simulink model "BaseEngineController_LS"  (Simulink 7.7)
settings: Solver=FixedStepDiscrete  StartTime=0.0  StopTime=10.0  RelTol=1e-3
PreLoadFcn:
  | try, eval([bdroot '_setup']); catch, eval('model_setup', ''); end
InitFcn:
  | try, eval([bdroot '_setup']); catch, eval('model_setup', ''); end
undefined symbols (not defined in the file): ECU555, High, motohawk_build_version, motohawk_trunc_name, motohawk_vardec_config_group, motohawk_vardec_path, True
libraries: MotoHawk_lib x1418, motohawk_control_primitives_lib x183, motohawk_engine_lib x32, simulink x21, motohawk_annotations_lib x9, AutoDoc_lib x8, simulink_extras x4, motohawk_ccp_examples_lib x1, motohawk_control_primitives_motoshare_lib x1
(part 12 of 27)

== system BaseEngineController_LS/Foreground/Control/Controller/Run/AC Control ==
  Sensors : Inport
  Trigger : TriggerPort  TriggerType=function-call
  AC Comp High Pressure : Subsystem  AncestorBlock=motohawk_control_primitives_lib/Hysterisis
      mask Display:
      | patch([0 0 1 1], [0 0.075 0.075 0], [230/255 0/255 0/255])
      | patch([0 0 1 1], [0.025 0.05 0.05 0.025], [150/255 0/255 0/255])
      | patch([0 0 1 1], [0 0.025 0.025 0], [0/255 0/255 0/255])
      | 
      | disp('HYSTERISIS')
  AC Comp Low Pressure : Subsystem  AncestorBlock=motohawk_control_primitives_lib/Hysterisis
      mask Display:
      | patch([0 0 1 1], [0 0.075 0.075 0], [230/255 0/255 0/255])
      | patch([0 0 1 1], [0.025 0.05 0.05 0.025], [150/255 0/255 0/255])
      | patch([0 0 1 1], [0 0.025 0.025 0], [0/255 0/255 0/255])
      | 
      | disp('HYSTERISIS')
  AC Comp Overspeed : Subsystem  AncestorBlock=motohawk_control_primitives_lib/Hysterisis
      mask Display:
      | patch([0 0 1 1], [0 0.075 0.075 0], [230/255 0/255 0/255])
      | patch([0 0 1 1], [0.025 0.05 0.05 0.025], [150/255 0/255 0/255])
      | patch([0 0 1 1], [0 0.025 0.025 0], [0/255 0/255 0/255])
      | 
      | disp('HYSTERISIS')
  AC Comp Overspeed1 : Subsystem  AncestorBlock=motohawk_control_primitives_lib/Hysterisis
      mask Display:
      | patch([0 0 1 1], [0 0.075 0.075 0], [230/255 0/255 0/255])
      | patch([0 0 1 1], [0.025 0.05 0.05 0.025], [150/255 0/255 0/255])
      | patch([0 0 1 1], [0 0.025 0.025 0], [0/255 0/255 0/255])
      | 
      | disp('HYSTERISIS')
  AC Comp Underspeed : Subsystem  AncestorBlock=motohawk_control_primitives_lib/Hysterisis
      mask Display:
      | patch([0 0 1 1], [0 0.075 0.075 0], [230/255 0/255 0/255])
      | patch([0 0 1 1], [0.025 0.05 0.05 0.025], [150/255 0/255 0/255])
      | patch([0 0 1 1], [0 0.025 0.025 0], [0/255 0/255 0/255])
      | 
      | disp('HYSTERISIS')
  AC Evap Temp Hyst : Subsystem  AncestorBlock=motohawk_control_primitives_lib/Hysterisis
      mask Display:
      | patch([0 0 1 1], [0 0.075 0.075 0], [230/255 0/255 0/255])
      | patch([0 0 1 1], [0.025 0.05 0.05 0.025], [150/255 0/255 0/255])
      | patch([0 0 1 1], [0 0.025 0.025 0], [0/255 0/255 0/255])
      | 
      | disp('HYSTERISIS')
  Bus Selector : BusSelector  OutputSignals=Raw.Digital.ACSw,Raw.NonLinearSensors.EVAP
  Bus Selector1 : BusSelector  OutputSignals=Raw.RPM
  Bus Selector2 : BusSelector  OutputSignals=RawProcessed.TPS
  Bus Selector3 : BusSelector  OutputSignals=Raw.LinearSensors.ACPres
  Bus Selector4 : BusSelector  OutputSignals=RawProcessed.TimeSinceRun
  Data Type Conversion : DataTypeConversion  OutDataTypeStr=uint16
  Data Type Conversion1 : DataTypeConversion  OutDataTypeStr=uint16
  Data Type Conversion2 : DataTypeConversion  OutDataTypeStr=uint16
  Logical Operator : Logic  Inputs=8  AllPortsSameDT=off  OutDataTypeStr=boolean
  Logical Operator{1..2,4,6} (4 alike) : Logic  Operator=NOT  AllPortsSameDT=off  OutDataTypeStr=boolean
  Logical Operator3 : Logic  AllPortsSameDT=off  OutDataTypeStr=boolean
  Relational Operator : RelationalOperator  OutDataTypeStr=boolean
  motohawk_calibration : MotoHawk_lib/Calibration & Probing Blocks/motohawk_calibration  nam='ACTempOn'  val=0  storage=Calibration  show_more=on  name_source=Use Parameter  data_type=double  read_level=1  write_level=1  ovr_cals=on  view_as=Number  enum_struct={'Disabled', 'Enabled'}  vector_style=Wide Row  use_help_units=off  help=''  units=''  use_header_enum=off  row_header_enum={}  col_header_enum={}  use_min_max=off  min_val=-inf  max_val=inf  use_precision=off  precision=''  gain=1  offset=0  exp=1  use_mototune_group=off  mototune_group=motohawk_vardec_path(gcb)
  motohawk_calibration1 : MotoHawk_lib/Calibration & Probing Blocks/motohawk_calibration  nam='ACSpdSlowOff'  val=200  storage=Calibration  show_more=on  name_source=Use Parameter  data_type=uint16  read_level=1  write_level=1  ovr_cals=on  view_as=Number  enum_struct={'Disabled', 'Enabled'}  vector_style=Wide Row  use_help_units=on  help='Engine speed at which the compressor turns off at low side'  units='RPM'  use_header_enum=off  row_header_enum={}  col_header_enum={}  use_min_max=off  min_val=-inf  max_val=inf  use_precision=off  precision=''  gain=1  offset=0  exp=1  use_mototune_group=off  mototune_group=motohawk_vardec_path(gcb)
  motohawk_calibration10 : MotoHawk_lib/Calibration & Probing Blocks/motohawk_calibration  nam='ACLowPresOff'  val=0  storage=Calibration  show_more=on  name_source=Use Parameter  data_type=uint16  read_level=1  write_level=1  ovr_cals=on  view_as=Number  enum_struct={'Disabled', 'Enabled'}  vector_style=Wide Row  use_help_units=off  help=''  units=''  use_header_enum=off  row_header_enum={}  col_header_enum={}  use_min_max=off  min_val=-inf  max_val=inf  use_precision=off  precision=''  gain=1  offset=0  exp=1  use_mototune_group=off  mototune_group=motohawk_vardec_path(gcb)
  motohawk_calibration11 : MotoHawk_lib/Calibration & Probing Blocks/motohawk_calibration  nam='ACHighPresOff'  val=0  storage=Calibration  show_more=on  name_source=Use Parameter  data_type=uint16  read_level=1  write_level=1  ovr_cals=on  view_as=Number  enum_struct={'Disabled', 'Enabled'}  vector_style=Wide Row  use_help_units=off  help=''  units=''  use_header_enum=off  row_header_enum={}  col_header_enum={}  use_min_max=off  min_val=-inf  max_val=inf  use_precision=off  precision=''  gain=1  offset=0  exp=1  use_mototune_group=off  mototune_group=motohawk_vardec_path(gcb)
  motohawk_calibration12 : MotoHawk_lib/Calibration & Probing Blocks/motohawk_calibration  nam='ACHighPresOn'  val=0  storage=Calibration  show_more=on  name_source=Use Parameter  data_type=uint16  read_level=1  write_level=1  ovr_cals=on  view_as=Number  enum_struct={'Disabled', 'Enabled'}  vector_style=Wide Row  use_help_units=off  help=''  units=''  use_header_enum=off  row_header_enum={}  col_header_enum={}  use_min_max=off  min_val=-inf  max_val=inf  use_precision=off  precision=''  gain=1  offset=0  exp=1  use_mototune_group=off  mototune_group=motohawk_vardec_path(gcb)
  motohawk_calibration2 : MotoHawk_lib/Calibration & Probing Blocks/motohawk_calibration  nam='ACSpdSlowOn'  val=400  storage=Calibration  show_more=on  name_source=Use Parameter  data_type=uint16  read_level=1  write_level=1  ovr_cals=on  view_as=Number  enum_struct={'Disabled', 'Enabled'}  vector_style=Wide Row  use_help_units=on  help='Engine speed at which the compressor turns on at low side'  units='RPM'  use_header_enum=off  row_header_enum={}  col_header_enum={}  use_min_max=off  min_val=-inf  max_val=inf  use_precision=off  precision=''  gain=1  offset=0  exp=1  use_mototune_group=off  mototune_group=motohawk_vardec_path(gcb)
  motohawk_calibration3 : MotoHawk_lib/Calibration & Probing Blocks/motohawk_calibration  nam='ACSpdFastOff'  val=4500  storage=Calibration  show_more=on  name_source=Use Parameter  data_type=uint16  read_level=1  write_level=1  ovr_cals=on  view_as=Number  enum_struct={'Disabled', 'Enabled'}  vector_style=Wide Row  use_help_units=on  help='Engine speed at which the compressor turns off at high side'  units='RPM'  use_header_enum=off  row_header_enum={}  col_header_enum={}  use_min_max=off  min_val=-inf  max_val=inf  use_precision=off  precision=''  gain=1  offset=0  exp=1  use_mototune_group=off  mototune_group=motohawk_vardec_path(gcb)
  motohawk_calibration4 : MotoHawk_lib/Calibration & Probing Blocks/motohawk_calibration  nam='ACSpdFastOn'  val=3000  storage=Calibration  show_more=on  name_source=Use Parameter  data_type=uint16  read_level=1  write_level=1  ovr_cals=on  view_as=Number  enum_struct={'Disabled', 'Enabled'}  vector_style=Wide Row  use_help_units=on  help='Engine speed at which the compressor turns on at high side'  units='RPM'  use_header_enum=off  row_header_enum={}  col_header_enum={}  use_min_max=off  min_val=-inf  max_val=inf  use_precision=off  precision=''  gain=1  offset=0  exp=1  use_mototune_group=off  mototune_group=motohawk_vardec_path(gcb)
  motohawk_calibration5 : MotoHawk_lib/Calibration & Probing Blocks/motohawk_calibration  nam='AC_TPSOff'  val=90  storage=Calibration  show_more=on  name_source=Use Parameter  data_type=uint16  read_level=1  write_level=1  ovr_cals=on  view_as=Number  enum_struct={'Disabled', 'Enabled'}  vector_style=Wide Row  use_help_units=on  help='Throttle position at which AC gets disengaged'  units='%'  use_header_enum=off  row_header_enum={}  col_header_enum={}  use_min_max=off  min_val=-inf  max_val=inf  use_precision=off  precision=''  gain=1  offset=0  exp=1  use_mototune_group=off  mototune_group=motohawk_vardec_path(gcb)
  motohawk_calibration6 : MotoHawk_lib/Calibration & Probing Blocks/motohawk_calibration  nam='AC_TPSOn'  val=80  storage=Calibration  show_more=on  name_source=Use Parameter  data_type=uint16  read_level=1  write_level=1  ovr_cals=on  view_as=Number  enum_struct={'Disabled', 'Enabled'}  vector_style=Wide Row  use_help_units=on  help='Throttle position at which AC gets engaged'  units='%'  use_header_enum=off  row_header_enum={}  col_header_enum={}  use_min_max=off  min_val=-inf  max_val=inf  use_precision=off  precision=''  gain=1  offset=0  exp=1  use_mototune_group=off  mototune_group=motohawk_vardec_path(gcb)
  motohawk_calibration7 : MotoHawk_lib/Calibration & Probing Blocks/motohawk_calibration  nam='ACTimeFromStartDelay'  val=3  storage=Calibration  show_more=on  name_source=Use Parameter  data_type=Inherit from 'Default Value'  read_level=1  write_level=1  ovr_cals=on  view_as=Number  enum_struct={'Disabled', 'Enabled'}  vector_style=Wide Row  use_help_units=on  help='Time from start AC enable delay'  units='Seconds'  use_header_enum=off  row_header_enum={}  col_header_enum={}  use_min_max=on  min_val=0  max_val=inf  use_precision=off  precision=''  gain=1  offset=0  exp=1  use_mototune_group=off  mototune_group=motohawk_vardec_path(gcb)
  motohawk_calibration8 : MotoHawk_lib/Calibration & Probing Blocks/motohawk_calibration  nam='ACTempOff'  val=0  storage=Calibration  show_more=on  name_source=Use Parameter  data_type=double  read_level=1  write_level=1  ovr_cals=on  view_as=Number  enum_struct={'Disabled', 'Enabled'}  vector_style=Wide Row  use_help_units=off  help=''  units=''  use_header_enum=off  row_header_enum={}  col_header_enum={}  use_min_max=off  min_val=-inf  max_val=inf  use_precision=off  precision=''  gain=1  offset=0  exp=1  use_mototune_group=off  mototune_group=motohawk_vardec_path(gcb)
  motohawk_calibration9 : MotoHawk_lib/Calibration & Probing Blocks/motohawk_calibration  nam='ACLowPresOn'  val=0  storage=Calibration  show_more=on  name_source=Use Parameter  data_type=uint16  read_level=1  write_level=1  ovr_cals=on  view_as=Number  enum_struct={'Disabled', 'Enabled'}  vector_style=Wide Row  use_help_units=off  help=''  units=''  use_header_enum=off  row_header_enum={}  col_header_enum={}  use_min_max=off  min_val=-inf  max_val=inf  use_precision=off  precision=''  gain=1  offset=0  exp=1  use_mototune_group=off  mototune_group=motohawk_vardec_path(gcb)
  motohawk_fault_action : MotoHawk_lib/Fault Management Blocks/motohawk_fault_action  nam='DisableAC'  output_status=on  eval_nam=DisableAC
  motohawk_probe1 : MotoHawk_lib/Calibration & Probing Blocks/motohawk_probe  nam='ACTempEnbl'  show_more=off  name_source=Use Parameter  read_level=1  view_as=Number  enum_struct={'Disabled', 'Enabled'}  vector_style=Wide Row  use_help_units=off  help=''  units=''  use_header_enum=off  row_header_enum={}  col_header_enum={}  use_precision=off  precision=''  gain=1  offset=0  exp=1  use_mototune_group=off  mototune_group=motohawk_vardec_path(gcb)
  motohawk_probe2 : MotoHawk_lib/Calibration & Probing Blocks/motohawk_probe  nam='ACRpmLowEnbl'  show_more=off  name_source=Use Parameter  read_level=1  view_as=Number  enum_struct={'Disabled', 'Enabled'}  vector_style=Wide Row  use_help_units=off  help=''  units=''  use_header_enum=off  row_header_enum={}  col_header_enum={}  use_precision=off  precision=''  gain=1  offset=0  exp=1  use_mototune_group=off  mototune_group=motohawk_vardec_path(gcb)
  motohawk_probe3 : MotoHawk_lib/Calibration & Probing Blocks/motohawk_probe  nam='ACRpmHighEnbl'  show_more=off  name_source=Use Parameter  read_level=1  view_as=Number  enum_struct={'Disabled', 'Enabled'}  vector_style=Wide Row  use_help_units=off  help=''  units=''  use_header_enum=off  row_header_enum={}  col_header_enum={}  use_precision=off  precision=''  gain=1  offset=0  exp=1  use_mototune_group=off  mototune_group=motohawk_vardec_path(gcb)
  motohawk_probe4 : MotoHawk_lib/Calibration & Probing Blocks/motohawk_probe  nam='ACTpsEnble'  show_more=off  name_source=Use Parameter  read_level=1  view_as=Number  enum_struct={'Disabled', 'Enabled'}  vector_style=Wide Row  use_help_units=off  help=''  units=''  use_header_enum=off  row_header_enum={}  col_header_enum={}  use_precision=off  precision=''  gain=1  offset=0  exp=1  use_mototune_group=off  mototune_group=motohawk_vardec_path(gcb)
  motohawk_probe5 : MotoHawk_lib/Calibration & Probing Blocks/motohawk_probe  nam='ACOutput'  show_more=off  name_source=Use Parameter  read_level=1  view_as=Number  enum_struct={'Disabled', 'Enabled'}  vector_style=Wide Row  use_help_units=off  help=''  units=''  use_header_enum=off  row_header_enum={}  col_header_enum={}  use_precision=off  precision=''  gain=1  offset=0  exp=1  use_mototune_group=off  mototune_group=motohawk_vardec_path(gcb)
  motohawk_probe6 : MotoHawk_lib/Calibration & Probing Blocks/motohawk_probe  nam='ACLowChrg'  show_more=off  name_source=Use Parameter  read_level=1  view_as=Number  enum_struct={'Disabled', 'Enabled'}  vector_style=Wide Row  use_help_units=off  help=''  units=''  use_header_enum=off  row_header_enum={}  col_header_enum={}  use_precision=off  precision=''  gain=1  offset=0  exp=1  use_mototune_group=off  mototune_group=motohawk_vardec_path(gcb)
  motohawk_probe7 : MotoHawk_lib/Calibration & Probing Blocks/motohawk_probe  nam='ACOverPressure'  show_more=off  name_source=Use Parameter  read_level=1  view_as=Number  enum_struct={'Disabled', 'Enabled'}  vector_style=Wide Row  use_help_units=off  help=''  units=''  use_header_enum=off  row_header_enum={}  col_header_enum={}  use_precision=off  precision=''  gain=1  offset=0  exp=1  use_mototune_group=off  mototune_group=motohawk_vardec_path(gcb)
  AC : Outport
  wires:
  Sensors/1 -> Bus Selector/1, Bus Selector1/1, Bus Selector2/1, Bus Selector3/1, Bus Selector4/1
  Logical Operator/1 -> motohawk_probe5/1, AC/1
  Bus Selector/1 -> Logical Operator/1  "<ACSw>"
  motohawk_calibration/1 -> AC Evap Temp Hyst/1(HiThresh)
  motohawk_calibration8/1 -> AC Evap Temp Hyst/2(LowThresh)
  AC Evap Temp Hyst/1(Threshold) -> motohawk_probe1/1, Logical Operator/2
  Bus Selector1/1 -> Data Type Conversion/1  "<RPM>"
  motohawk_calibration1/1 -> AC Comp Underspeed/2(LowThresh)
  motohawk_calibration2/1 -> AC Comp Underspeed/1(HiThresh)
  AC Comp Overspeed/1(Threshold) -> Logical Operator2/1
  motohawk_calibration4/1 -> AC Comp Overspeed/2(LowThresh)
  motohawk_calibration3/1 -> AC Comp Overspeed/1(HiThresh)
  AC Comp Underspeed/1(Threshold) -> Logical Operator3/1, motohawk_probe2/1
  Logical Operator2/1 -> Logical Operator3/2, motohawk_probe3/1
  Logical Operator3/1 -> Logical Operator/3
  Bus Selector2/1 -> Data Type Conversion2/1  "<TPS>"
  motohawk_calibration5/1 -> AC Comp Overspeed1/1(HiThresh)
  motohawk_calibration6/1 -> AC Comp Overspeed1/2(LowThresh)
  AC Comp Overspeed1/1(Threshold) -> Logical Operator4/1
  Logical Operator4/1 -> Logical Operator/4, motohawk_probe4/1
  Bus Selector3/1 -> Data Type Conversion1/1  "<ACPres>"
  motohawk_calibration9/1 -> AC Comp Low Pressure/1(HiThresh)
  motohawk_calibration10/1 -> AC Comp Low Pressure/2(LowThresh)
  motohawk_calibration11/1 -> AC Comp High Pressure/1(HiThresh)
  motohawk_calibration12/1 -> AC Comp High Pressure/2(LowThresh)
  AC Comp High Pressure/1(Threshold) -> Logical Operator1/1
  AC Comp Low Pressure/1(Threshold) -> motohawk_probe6/1, Logical Operator/5
  Logical Operator1/1 -> motohawk_probe7/1, Logical Operator/6
  motohawk_fault_action/1 -> Logical Operator6/1
  Logical Operator6/1 -> Logical Operator/8
  Bus Selector4/1 -> Relational Operator/1  "<TimeSinceRun>"
  motohawk_calibration7/1 -> Relational Operator/2
  Relational Operator/1 -> Logical Operator/7
  Bus Selector/2 -> AC Evap Temp Hyst/3(Signal)  "<EVAP>"
  Data Type Conversion/1 -> AC Comp Underspeed/3(Signal), AC Comp Overspeed/3(Signal)
  Data Type Conversion1/1 -> AC Comp Low Pressure/3(Signal), AC Comp High Pressure/3(Signal)
  Data Type Conversion2/1 -> AC Comp Overspeed1/3(Signal)

== system BaseEngineController_LS/Foreground/Control/Controller/Run/AirFlow Manager ==
  MinGovInfo : Inport
  MaxGovInfo : Inport  Port=2
  Sensors : Inport  Port=3
  Bus Selector1 : BusSelector  OutputSignals=RawIndexes.RPM09Idx
  Bus Selector2 : BusSelector  OutputSignals=Raw.PotSensors.APP1
  Bus Selector3 : BusSelector  OutputSignals=MaxGovPID,MaxGovState
  Bus Selector4 : BusSelector  OutputSignals=OnIdle,BaseAirOfst,MinGovAirPID
  Bus Selector7 : BusSelector  OutputSignals=RawProcessed.ETCRequest
  Logical Operator : Logic  Operator=NOT  AllPortsSameDT=off  OutDataTypeStr=boolean
  Multiport Switch : MultiPortSwitch  DataPortOrder=Zero-based contiguous  Inputs=2  zeroidx=on
  Saturation : motohawk_control_primitives_lib/Saturation  SystemSampleTime=-1
  ShutDownTasksComplete Reset : Subsystem  TreatAsAtomicUnit=on
  Sum1 : Sum
  Sum2 : Sum
  Switch1 : Switch  Threshold=0.5
  Switch2 : Switch  Threshold=1
  Switch4 : Switch  Threshold=1
  motohawk_calibration : MotoHawk_lib/Calibration & Probing Blocks/motohawk_calibration  nam='IACTypeCal'  val=0  storage=Calibration  show_more=on  name_source=Use Parameter  data_type=uint8  read_level=1  write_level=1  ovr_cals=on  view_as=Enumeration  enum_struct={'2-Wire', '3-Wire'}  vector_style=Wide Row  use_help_units=off  help=''  units=''  use_header_enum=off  row_header_enum={}  col_header_enum={}  use_min_max=off  min_val=-inf  max_val=inf  use_precision=off  precision=''  gain=1  offset=0  exp=1  use_mototune_group=off  mototune_group=motohawk_vardec_path(gcb)
  motohawk_calibration1 : MotoHawk_lib/Calibration & Probing Blocks/motohawk_calibration  nam='ThrottleSource'  val=1  storage=Calibration  show_more=on  name_source=Use Parameter  data_type=boolean  read_level=1  write_level=1  ovr_cals=on  view_as=Enumeration  enum_struct={'APP1', 'NORMAL'}  vector_style=Wide Row  use_help_units=on  help='Selects source of throttle command'  units=''  use_header_enum=off  row_header_enum={}  col_header_enum={}  use_min_max=off  min_val=-inf  max_val=inf  use_precision=off  precision=''  gain=1  offset=0  exp=1  use_mototune_group=on  mototune_group=motohawk_vardec_path(gcb)
  motohawk_calibration2 : MotoHawk_lib/Calibration & Probing Blocks/motohawk_calibration  nam='AirControlSource'  val=0  storage=Calibration  show_more=on  name_source=Use Parameter  data_type=boolean  read_level=1  write_level=1  ovr_cals=on  view_as=Enumeration  enum_struct={'ETC', 'IAC'}  vector_style=Wide Row  use_help_units=on  help='Selects source of idle air control'  units=''  use_header_enum=off  row_header_enum={}  col_header_enum={}  use_min_max=off  min_val=-inf  max_val=inf  use_precision=off  precision=''  gain=1  offset=0  exp=1  use_mototune_group=on  mototune_group=motohawk_vardec_path(gcb)
  motohawk_data_def : MotoHawk_lib/Data Storage Blocks/motohawk_data_def  nam='IACType'  container_nam=''  data=0  typ=uint8  struct_nam='MyStruct'  storage=NonVolatile  outputRef=off  use_vardec=off  window=Calibration  read_level=1  write_level=1  ovr_cals=on  view_as=Enumeration  enum_struct={'2-Wire', '3-Wire'}  vector_style=Wide Row  use_help_units=on  help='IAC type if being used'  units=''  use_header_enum=off  row_header_enum=''  col_header_enum=''  use_min_max=off  min_val=-inf  max_val=inf  use_precision=off  precision=''  gain=1  offset=0  exp=1  use_mototune_group=on  mototune_group=motohawk_vardec_path(gcb)  eval_name=MyData  data_stores=motohawk_sfun_data_def_data_stores  struct_instances=motohawk_sfun_data_def_struct_instances  vardecs=motohawk_sfun_data_def_vardecs
  motohawk_data_write : MotoHawk_lib/Data Storage Blocks/motohawk_data_write  source=Lookup By Name  structure=Scalar  operation=Write entire data structure at once  sz_vec=9  sz_row=2  sz_col=9  typ=uint8  nam='IACType'  checkNull=on  write_read_only=off  struct_inst_name=''  struct_name='MyStruct'
  motohawk_interpolation_1d1 : MotoHawk_lib/Lookup Tables/motohawk_interpolation_1d  nam='MinETCSetPtLimit'  table_data=[0 0 0 0 0 0 0 0 0]  show_more=on  data_type=Inherit from 'Table Data'  storage=NonAdaptive  read_level=1  write_level=1  ovr_cals=on  use_help=on  help='Min allowable ETC position.'  units='%'  use_min_max=on  min_val=0  max_val=100  use_precision=off  precision=''  gain=1  offset=0  exp=1  use_links=off  prelookup_block=''  output_name=''  use_mototune_group=on  mototune_group=motohawk_vardec_path(gcb)
  motohawk_interpolation_1d2 : MotoHawk_lib/Lookup Tables/motohawk_interpolation_1d  nam='MaxETCSetPtLimit'  table_data=[60 70 70 70 75 85 92 100 100]  show_more=on  data_type=Inherit from 'Table Data'  storage=NonAdaptive  read_level=1  write_level=1  ovr_cals=on  use_help=on  help='Maximum allowable ETC position.'  units='%'  use_min_max=on  min_val=0  max_val=100  use_precision=off  precision=''  gain=1  offset=0  exp=1  use_links=off  prelookup_block=''  output_name=''  use_mototune_group=on  mototune_group=motohawk_vardec_path(gcb)
  motohawk_probe1 : MotoHawk_lib/Calibration & Probing Blocks/motohawk_probe  nam='ETCRequestFinal'  show_more=on  name_source=Use Parameter  read_level=1  view_as=Number  enum_struct={'Disabled', 'Enabled'}  vector_style=Wide Row  use_help_units=on  help='Final ETC request sent to ETC controller from Run state.'  units='%'  use_header_enum=off  row_header_enum={}  col_header_enum={}  use_precision=on  precision='5.2'  gain=1  offset=0  exp=1  use_mototune_group=on  mototune_group=motohawk_vardec_path(gcb)
  ETC% : Outport
  wires:
  Logical Operator/1 -> Switch4/2
  Bus Selector4/1 -> Logical Operator/1  "<OnIdle>"
  Bus Selector4/3 -> Sum2/2  "<MinGovAirPID>"
  Bus Selector4/2 -> Sum2/1, Sum1/2  "<BaseAirOfst>"
  Sum2/1 -> Multiport Switch/3, Switch4/3
  Sum1/1 -> Switch4/1
  Bus Selector7/1 -> Sum1/1  "<ETCRequest>"
  MinGovInfo/1 -> Bus Selector4/1
  Bus Selector3/2 -> Switch2/2  "<MaxGovState>"
  Bus Selector3/1 -> Switch2/1  "<MaxGovPID>"
  MaxGovInfo/1 -> Bus Selector3/1
  Bus Selector2/1 -> Switch1/3  "<APP1>"
  motohawk_calibration1/1 -> Switch1/2
  Switch2/1 -> Saturation/1
  motohawk_interpolation_1d1/1 -> Saturation/2
  Sensors/1 -> Bus Selector7/1, Bus Selector1/1, Bus Selector2/1
  motohawk_interpolation_1d2/1 -> Saturation/3
  Saturation/1 -> Switch1/1
  Bus Selector1/1 -> motohawk_interpolation_1d2/1, motohawk_interpolation_1d1/1  "<RPM09Idx>"
  motohawk_calibration2/1 -> Multiport Switch/1, ShutDownTasksComplete Reset/Enable
  Multiport Switch/1 -> ETC%/1, motohawk_probe1/1
  Switch1/1 -> Multiport Switch/2
  motohawk_calibration/1 -> motohawk_data_write/1
  Switch4/1 -> Switch2/3

== system BaseEngineController_LS/Foreground/Control/Controller/Run/Base Equiv Ratio ==
  Sensors : Inport
  Bus Creator : BusCreator  Inputs=5
  Bus Selector : BusSelector  OutputSignals=RawIndexes.MAP17Idx,RawIndexes.RPM17Idx
  Bus Selector1 : BusSelector  OutputSignals=VirtualIndexes.TimeSinceRun09,RawIndexes.ECT05Idx
  Bus Selector2 : BusSelector  OutputSignals=RawIndexes.MAP05Idx,RawIndexes.ECT09Idx
  Bus Selector4 : BusSelector  OutputSignals=RawIndexes.MAP05Idx,RawIndexes.IAT05Idx
  Bus Selector5 : BusSelector  OutputSignals=RawProcessed.TimeSinceRun
  Bus Selector6 : BusSelector  OutputSignals=RawIndexes.MAP05Idx,RawIndexes.CAT05Idx
  MinMax : MinMax  Function=max  Inputs=5
  Warm Up Fuel Holdoff : Subsystem
  motohawk_interpolation_2d1 : MotoHawk_lib/Lookup Tables/motohawk_interpolation_2d  nam='WarmUpEqRatio'  table_data=ones(5,9)  show_more=on  data_type=Inherit from 'Table Data'  storage=NonAdaptive  read_level=1  write_level=1  ovr_cals=on  use_help=on  help='Requested eq. ratio as a function of ECT and MAP.'  units='phi'  use_min_max=on  min_val=0  max_val=10  use_precision=on  precision=''  gain=1  offset=0  exp=1  use_links=off  row_prelookup_block=''  col_prelookup_block=''  output_name=''  use_mototune_group=on  mototune_group=motohawk_vardec_path(gcb)
  motohawk_interpolation_2d2 : MotoHawk_lib/Lookup Tables/motohawk_interpolation_2d  nam='WarmUpTimeRatio'  table_data=ones(9,5)  show_more=on  data_type=Inherit from 'Table Data'  storage=NonAdaptive  read_level=1  write_level=1  ovr_cals=on  use_help=on  help='Requested eq. ratio as a function of TimeSinceRun and ECT. Use for cold temps'  units='phi'  use_min_max=on  min_val=0  max_val=10  use_precision=on  precision=''  gain=1  offset=0  exp=1  use_links=off  row_prelookup_block=''  col_prelookup_block=''  output_name=''  use_mototune_group=on  mototune_group=motohawk_vardec_path(gcb)
  motohawk_interpolation_2d3 : MotoHawk_lib/Lookup Tables/motohawk_interpolation_2d  nam='DesEquivRatio'  table_data=ones(17)  show_more=on  data_type=Inherit from 'Table Data'  storage=NonAdaptive  read_level=1  write_level=1  ovr_cals=on  use_help=on  help='Desired liquid equivalence ratio.'  units=''  use_min_max=on  min_val=0  max_val=inf  use_precision=on  precision=''  gain=1  offset=0  exp=1  use_links=off  row_prelookup_block=''  col_prelookup_block=''  output_name=''  use_mototune_group=on  mototune_group=motohawk_vardec_path(gcb)
  motohawk_interpolation_2d5 : MotoHawk_lib/Lookup Tables/motohawk_interpolation_2d  nam='IntakeAirTempEnrichment'  table_data=ones(5,5)  show_more=on  data_type=Inherit from 'Table Data'  storage=NonAdaptive  read_level=1  write_level=1  ovr_cals=on  use_help=on  help='Requested on base eq. ratio as a function of IAT and MAP'  units='phi'  use_min_max=on  min_val=0  max_val=10  use_precision=on  precision=''  gain=1  offset=0  exp=1  use_links=off  row_prelookup_block=''  col_prelookup_block=''  output_name=''  use_mototune_group=on  mototune_group=motohawk_vardec_path(gcb)
  motohawk_interpolation_2d6 : MotoHawk_lib/Lookup Tables/motohawk_interpolation_2d  nam='ChargeAirTempEnrichment'  table_data=ones(5,5)  show_more=on  data_type=Inherit from 'Table Data'  storage=NonAdaptive  read_level=1  write_level=1  ovr_cals=on  use_help=on  help='Requsted base eq. ratio as a function of CAT and MAP'  units='phi'  use_min_max=off  min_val=0  max_val=inf  use_precision=on  precision=''  gain=1  offset=0  exp=1  use_links=off  row_prelookup_block=''  col_prelookup_block=''  output_name=''  use_mototune_group=on  mototune_group=motohawk_vardec_path(gcb)
  motohawk_override_abs : MotoHawk_lib/Calibration & Probing Blocks/motohawk_override_abs  SystemSampleTime=-1  parent_name='EquivRatio'  parent_val=0  show_more=on  name_source=Use Parameter  parent_read_level=1  parent_override_level=1  view_as=Number  enum_struct={'Disabled', 'Enabled'}  use_help_units=off  parent_help=''  parent_units=''  use_min_max=off  parent_min=-inf  parent_max=inf  use_precision=off  parent_precision=''  parent_gain=1  parent_offset=0  parent_exp=1  use_mototune_group=on  parent_group=motohawk_vardec_path(gcb)
  motohawk_probe : MotoHawk_lib/Calibration & Probing Blocks/motohawk_probe  nam='BaseEquivRatio'  show_more=on  name_source=Use Parameter  read_level=1  view_as=Number  enum_struct={'Disabled', 'Enabled'}  vector_style=Wide Row  use_help_units=on  help='Base equivalence ratio for selected fuel system.'  units=''  use_header_enum=off  row_header_enum={}  col_header_enum={}  use_precision=on  precision=''  gain=1  offset=0  exp=1  use_mototune_group=on  mototune_group=motohawk_vardec_path(gcb)
  EquivRatioInfo : Outport
  wires:
  Bus Selector/2 -> motohawk_interpolation_2d3/2  "<RPM17Idx>"
  Bus Selector/1 -> motohawk_interpolation_2d3/1  "<MAP17Idx>"
  Sensors/1 -> Bus Selector/1, Bus Selector2/1, Bus Selector1/1, Bus Selector4/1, Bus Selector6/1, Bus Selector5/1
  Bus Selector2/1 -> motohawk_interpolation_2d1/1  "<MAP05Idx>"
  Bus Selector2/2 -> motohawk_interpolation_2d1/2  "<ECT09Idx>"
  Bus Creator/1 -> EquivRatioInfo/1
  MinMax/1 -> motohawk_probe/1, Bus Creator/1  "DesEquivRatio"
  motohawk_override_abs/1 -> MinMax/1
  motohawk_interpolation_2d3/1 -> motohawk_override_abs/1
  Bus Selector1/1 -> motohawk_interpolation_2d2/1  "<TimeSinceRun09>"
  Bus Selector1/2 -> motohawk_interpolation_2d2/2, Warm Up Fuel Holdoff/3(ECTIdx)  "<ECT05Idx>"
  Bus Selector4/1 -> motohawk_interpolation_2d5/1  "<MAP05Idx>"
  Bus Selector4/2 -> motohawk_interpolation_2d5/2  "<IAT05Idx>"
  motohawk_interpolation_2d5/1 -> Bus Creator/4, MinMax/4  "IATEnrichment"
  Warm Up Fuel Holdoff/1(Out1) -> Bus Creator/3, MinMax/3  "WarmUptimeRatio"
  motohawk_interpolation_2d2/1 -> Warm Up Fuel Holdoff/2(WarmuUpTimeRatio)  "WarmUptimeRatio"
  Bus Selector5/1 -> Warm Up Fuel Holdoff/1(TimeSinceRun)  "<TimeSinceRun>"
  Bus Selector6/1 -> motohawk_interpolation_2d6/1  "<MAP05Idx>"
  Bus Selector6/2 -> motohawk_interpolation_2d6/2  "<CAT05Idx>"
  motohawk_interpolation_2d6/1 -> Bus Creator/5, MinMax/5  "CATEnrichment"
  motohawk_interpolation_2d1/1 -> Bus Creator/2, MinMax/2  "WarmUpRatio"

== system BaseEngineController_LS/Foreground/Control/Controller/Run/Boost Control ==
  note: BOOST Level
  Sensors : Inport
  Trigger : TriggerPort  TriggerType=function-call
  BoostControl Adapt : Subsystem  TreatAsAtomicUnit=on
  Bus Selector : BusSelector  OutputSignals=RawIndexes.RPM09Idx
  Bus Selector1 : BusSelector  OutputSignals=Raw.LinearSensors.Map_Time,AirCalcs.Baro
  Bus Selector3 : BusSelector  OutputSignals=Raw.Digital.Scramble
  Bus Selector4 : BusSelector  OutputSignals=RawIndexes.SysVolt09Idx
  Bus Selector5 : BusSelector  OutputSignals=RawIndexes.VSPD09Idx
  Bus Selector6 : BusSelector  OutputSignals=RawIndexes.ECT05Idx,RawIndexes.IAT05Idx
  Constant : Constant  Value=0
  Logical Operator : Logic  Operator=NOT  AllPortsSameDT=off  OutDataTypeStr=boolean
  MinMax : MinMax  Inputs=2
  MinMax2 : MinMax  Inputs=2
  Product : Product  RndMeth=Zero
  Relational Operator : RelationalOperator  Operator=<  OutDataTypeStr=boolean
  Sum : Sum  Inputs=+++
  Sum1 : Sum  Inputs=+-
  Sum2 : Sum  Inputs=|++
  Sum3 : Sum  Inputs=|++
  Switch : Switch  Criteria=u2 > Threshold
  Unit Delay : UnitDelay  SampleTime=-1
  Universal PID (Tunable & Scheduled) : Subsystem  AncestorBlock=motohawk_control_primitives_lib/Universal PID (Tunable & Scheduled)  mask(Universal PID (Tunable)){nam='BoostCtl', prefix='BoostCtl', samp_time=-1, units='dutyCycle', group=motohawk_vardec_path(gcb)}
      mask prompts: nam "Name"; samp_time "Sample Time"; group "MotoTune Group String"
      mask help:
      | This block wraps a 'Universal PID' block to provide gain scheduling and calibrations and probes for most parameters.
      |
      | If 'Sample Time' is -1, then extra code and RAM will be generated to dynamically calculate dt.
      mask init:
      | grp = [group ' | ' nam];
      mask Display:
      | patch([0 0 1 1], [0 0.075 0.075 0], [230/255 0/255 0/255])
      | patch([0 0 1 1], [0.025 0.05 0.05 0.025], [150/255 0/255 0/255])
      | patch([0 0 1 1], [0 0.025 0.025 0], [0/255 0/255 0/255])
      | 
      | disp([nam '\n(PID w/ Gain Schedules)']);
  Variable Rate Limiter : motohawk_control_primitives_lib/Variable Rate Limiter  SystemSampleTime=-1
  kPa to PSI : Gain  Gain=0.145038
  motohawk_calibration : MotoHawk_lib/Calibration & Probing Blocks/motohawk_calibration  nam='BoostRiseRate'  val=8  storage=Calibration  show_more=on  name_source=Use Parameter  data_type=Inherit from 'Default Value'  read_level=1  write_level=1  ovr_cals=on  view_as=Number  enum_struct={'Disabled', 'Enabled'}  vector_style=Wide Row  use_help_units=on  help='Maximum rate boost builds at'  units='PSI/sec'  use_header_enum=off  row_header_enum={}  col_header_enum={}  use_min_max=on  min_val=0  max_val=10000  use_precision=off  precision=''  gain=1  offset=0  exp=1  use_mototune_group=off  mototune_group=motohawk_vardec_path(gcb)
  motohawk_calibration1 : MotoHawk_lib/Calibration & Probing Blocks/motohawk_calibration  nam='BoostFallRate'  val=-20  storage=Calibration  show_more=on  name_source=Use Parameter  data_type=Inherit from 'Default Value'  read_level=1  write_level=1  ovr_cals=on  view_as=Number  enum_struct={'Disabled', 'Enabled'}  vector_style=Wide Row  use_help_units=on  help='Maximum rate boost falls at'  units='PSI/sec'  use_header_enum=off  row_header_enum={}  col_header_enum={}  use_min_max=on  min_val=-10000  max_val=0  use_precision=off  precision=''  gain=1  offset=0  exp=1  use_mototune_group=off  mototune_group=motohawk_vardec_path(gcb)
  motohawk_calibration2 : MotoHawk_lib/Calibration & Probing Blocks/motohawk_calibration  nam='BoostActivationThreshold'  val=8  storage=Calibration  show_more=on  name_source=Use Parameter  data_type=Inherit from 'Default Value'  read_level=1  write_level=1  ovr_cals=on  view_as=Number  enum_struct={'Disabled', 'Enabled'}  vector_style=Wide Row  use_help_units=on  help='Minimum boost pressure before controller is activated, usually set to wastegate spring pressure'  units='PSI'  use_header_enum=off  row_header_enum={}  col_header_enum={}  use_min_max=off  min_val=-inf  max_val=inf  use_precision=off  precision=''  gain=1  offset=0  exp=1  use_mototune_group=off  mototune_group=motohawk_vardec_path(gcb)
  motohawk_calibration3 : MotoHawk_lib/Calibration & Probing Blocks/motohawk_calibration  nam='BoostScrambleAdder'  val=5  storage=Calibration  show_more=on  name_source=Use Parameter  data_type=Inherit from 'Default Value'  read_level=1  write_level=1  ovr_cals=on  view_as=Number  enum_struct={'Disabled', 'Enabled'}  vector_style=Wide Row  use_help_units=on  help='Amount of pressure to increase target by when scramble button is activated'  units='PSI'  use_header_enum=off  row_header_enum={}  col_header_enum={}  use_min_max=on  min_val=-100  max_val=100  use_precision=off  precision=''  gain=1  offset=0  exp=1  use_mototune_group=off  mototune_group=motohawk_vardec_path(gcb)
  motohawk_interpolation_1d : MotoHawk_lib/Lookup Tables/motohawk_interpolation_1d  nam='BoostECTLimit'  table_data=[0 0 0 0 0]  show_more=on  data_type=int8  storage=NonAdaptive  read_level=1  write_level=1  ovr_cals=on  use_help=on  help='Boost limit as a function of ECT'  units='PSI'  use_min_max=on  min_val=0  max_val=100  use_precision=off  precision=''  gain=1  offset=0  exp=1  use_links=off  prelookup_block=''  output_name=''  use_mototune_group=off  mototune_group=motohawk_vardec_path(gcb)
  motohawk_interpolation_1d2 : MotoHawk_lib/Lookup Tables/motohawk_interpolation_1d  nam='WGDeadTime'  table_data=[1.495 1.293 1.155 1.05 0.968 0.898 0.865 0.823 0.743]  show_more=on  data_type=Inherit from 'Table Data'  storage=NonAdaptive  read_level=1  write_level=1  ovr_cals=on  use_help=on  help='Wastegate turn on time'  units='ms'  use_min_max=on  min_val=0  max_val=1000  use_precision=off  precision='2.3'  gain=1  offset=0  exp=1  use_links=off  prelookup_block=''  output_name=''  use_mototune_group=on  mototune_group=motohawk_vardec_path(gcb)
  motohawk_interpolation_1d3 : MotoHawk_lib/Lookup Tables/motohawk_interpolation_1d  nam='BoostIATLimit'  table_data=[0 0 0 0 0]  show_more=on  data_type=int8  storage=NonAdaptive  read_level=1  write_level=1  ovr_cals=on  use_help=on  help='Boost limit as a function of IAT'  units='PSI'  use_min_max=on  min_val=0  max_val=100  use_precision=off  precision=''  gain=1  offset=0  exp=1  use_links=off  prelookup_block=''  output_name=''  use_mototune_group=off  mototune_group=motohawk_vardec_path(gcb)
  motohawk_interpolation_2d : MotoHawk_lib/Lookup Tables/motohawk_interpolation_2d  nam='BoostControlBase'  table_data=ones(9,9)  show_more=on  data_type=uint8  storage=NonAdaptive  read_level=1  write_level=1  ovr_cals=on  use_help=on  help='Base boost duty cycle table for feed forward'  units='dutyCycle'  use_min_max=on  min_val=0  max_val=100  use_precision=off  precision=''  gain=1  offset=0  exp=1  use_links=off  row_prelookup_block=''  col_prelookup_block=''  output_name=''  use_mototune_group=off  mototune_group=motohawk_vardec_path(gcb)
  motohawk_interpolation_2d1 : MotoHawk_lib/Lookup Tables/motohawk_interpolation_2d  nam='BoostControlBase_Adapt'  table_data=ones(9,9)  show_more=on  data_type=double  storage=Adaptive - NonVolatile  read_level=1  write_level=1  ovr_cals=on  use_help=on  help='Base boost duty cycle table for feed forward'  units='dutyCycle'  use_min_max=on  min_val=0  max_val=100  use_precision=off  precision=''  gain=1  offset=0  exp=1  use_links=off  row_prelookup_block=''  col_prelookup_block=''  output_name=''  use_mototune_group=off  mototune_group=motohawk_vardec_path(gcb)
  motohawk_interpolation_2d2 : MotoHawk_lib/Lookup Tables/motohawk_interpolation_2d  nam='BoostTarget'  table_data=ones(9,9)*15  show_more=on  data_type=int8  storage=NonAdaptive  read_level=1  write_level=1  ovr_cals=on  use_help=on  help='Target boost as a function of RPM and VSPD'  units='PSI'  use_min_max=on  min_val=0  max_val=100  use_precision=off  precision=''  gain=1  offset=0  exp=1  use_links=off  row_prelookup_block=''  col_prelookup_block=''  output_name=''  use_mototune_group=off  mototune_group=motohawk_vardec_path(gcb)
  motohawk_prelookup : MotoHawk_lib/Lookup Tables/motohawk_prelookup  nam='BoostTarget'  breakpoint_data=[0 5 10 15 20 25 30 35 40]  show_more=on  data_type=Inherit from 'Table Data'  storage=Constant  read_level=1  write_level=1  ovr_cals=on  use_help=off  help=''  units=''  use_min_max=on  min_val=0  max_val=inf  use_precision=off  precision=''  gain=1  offset=0  exp=1  use_links=off  input_name=''  use_mototune_group=off  mototune_group=motohawk_vardec_path(gcb)
  motohawk_probe : MotoHawk_lib/Calibration & Probing Blocks/motohawk_probe  nam='BoostControlPID_ITerm'  show_more=on  name_source=Use Parameter  read_level=1  view_as=Number  enum_struct={'Disabled', 'Enabled'}  vector_style=Wide Row  use_help_units=on  help='Boost controller PID I term'  units=''  use_header_enum=off  row_header_enum={}  col_header_enum={}  use_precision=off  precision=''  gain=1  offset=0  exp=1  use_mototune_group=off  mototune_group=motohawk_vardec_path(gcb)
  motohawk_probe1 : MotoHawk_lib/Calibration & Probing Blocks/motohawk_probe  nam='BoostControlPID'  show_more=on  name_source=Use Parameter  read_level=1  view_as=Number  enum_struct={'Disabled', 'Enabled'}  vector_style=Wide Row  use_help_units=on  help='Boost controller PID output'  units='dutyCycle'  use_header_enum=off  row_header_enum={}  col_header_enum={}  use_precision=off  precision=''  gain=1  offset=0  exp=1  use_mototune_group=off  mototune_group=motohawk_vardec_path(gcb)
  motohawk_probe2 : MotoHawk_lib/Calibration & Probing Blocks/motohawk_probe  nam='BoostControlTarget'  show_more=on  name_source=Use Parameter  read_level=1  view_as=Number  enum_struct={'Disabled', 'Enabled'}  vector_style=Wide Row  use_help_units=on  help='Final boost target'  units='PSI'  use_header_enum=off  row_header_enum={}  col_header_enum={}  use_precision=off  precision=''  gain=1  offset=0  exp=1  use_mototune_group=off  mototune_group=motohawk_vardec_path(gcb)
  motohawk_probe3 : MotoHawk_lib/Calibration & Probing Blocks/motohawk_probe  nam='BoostControlDutyCycleOut'  show_more=on  name_source=Use Parameter  read_level=1  view_as=Number  enum_struct={'Disabled', 'Enabled'}  vector_style=Wide Row  use_help_units=on  help='Boost controller final duty cycle out'  units='dutyCycle'  use_header_enum=off  row_header_enum={}  col_header_enum={}  use_precision=off  precision=''  gain=1  offset=0  exp=1  use_mototune_group=off  mototune_group=motohawk_vardec_path(gcb)
  motohawk_probe4 : MotoHawk_lib/Calibration & Probing Blocks/motohawk_probe  nam='BoostControlDutyCycleFF'  show_more=off  name_source=Use Parameter  read_level=1  view_as=Number  enum_struct={'Disabled', 'Enabled'}  vector_style=Wide Row  use_help_units=off  help=''  units=''  use_header_enum=off  row_header_enum={}  col_header_enum={}  use_precision=off  precision=''  gain=1  offset=0  exp=1  use_mototune_group=off  mototune_group=motohawk_vardec_path(gcb)
  Wastegate : Outport
  wires:
  Sensors/1 -> Bus Selector/1, Bus Selector1/1, Bus Selector3/1, Bus Selector6/1, Bus Selector4/1, Bus Selector5/1
  Bus Selector/1 -> motohawk_interpolation_2d/2, motohawk_interpolation_2d1/2, motohawk_interpolation_2d2/2  "<RPM09Idx>"
  motohawk_prelookup/1 -> motohawk_interpolation_2d/1, motohawk_interpolation_2d1/1
  Bus Selector1/1 -> Sum1/1  "<Map_Time>"
  Bus Selector1/2 -> Sum1/2  "<Baro>"
  Sum1/1 -> kPa to PSI/1
  kPa to PSI/1 -> Universal PID (Tunable & Scheduled)/1(Actual), Relational Operator/1
  motohawk_calibration/1 -> Variable Rate Limiter/2
  motohawk_calibration1/1 -> Variable Rate Limiter/3
  Variable Rate Limiter/1 -> Universal PID (Tunable & Scheduled)/2(SetPoint)
  Relational Operator/1 -> Universal PID (Tunable & Scheduled)/3(ResetAll), Switch/2, Logical Operator/1
  motohawk_calibration2/1 -> Relational Operator/2
  Constant/1 -> Switch/1
  Switch/1 -> Wastegate/1
  motohawk_interpolation_2d/1 -> Sum/2, motohawk_probe4/1
  Universal PID (Tunable & Scheduled)/1(MinGovOut) -> Sum/3, motohawk_probe1/1
  motohawk_interpolation_2d1/1 -> Sum/1
  Logical Operator/1 -> BoostControl Adapt/Enable, BoostControl Adapt/1(Active State)
  Universal PID (Tunable & Scheduled)/2(MinGovITerm) -> Unit Delay/1, motohawk_probe/1
  Unit Delay/1 -> BoostControl Adapt/2(ITerm)
  MinMax2/1 -> motohawk_prelookup/1, Variable Rate Limiter/1, motohawk_probe2/1
  motohawk_interpolation_2d2/1 -> Sum2/1
  Bus Selector3/1 -> Product/1  "<Scramble>"
  Product/1 -> Sum2/2
  motohawk_calibration3/1 -> Product/2
  Sum/1 -> Sum3/1
  Sum3/1 -> Switch/3, motohawk_probe3/1
  motohawk_interpolation_1d2/1 -> Sum3/2
  Bus Selector4/1 -> motohawk_interpolation_1d2/1  "<SysVolt09Idx>"
  Bus Selector5/1 -> motohawk_interpolation_2d2/1  "<VSPD09Idx>"
  Sum2/1 -> MinMax2/1
  Bus Selector6/1 -> motohawk_interpolation_1d/1  "<ECT05Idx>"
  Bus Selector6/2 -> motohawk_interpolation_1d3/1  "<IAT05Idx>"
  motohawk_interpolation_1d3/1 -> MinMax/2
  motohawk_interpolation_1d/1 -> MinMax/1
  MinMax/1 -> MinMax2/2

== system BaseEngineController_LS/Foreground/Control/Controller/Run/DFCO ==
  EquivRatioInfo : Inport
  Sensors : Inport  Port=2
  Trigger : TriggerPort  TriggerType=function-call
  Bus Creator : BusCreator  Inputs=5
  Bus Selector : BusSelector  OutputSignals=DesEquivRatio,WarmUpRatio,WarmUptimeRatio,IATEnrichment,CATEnrichment
  DesEquivRatioMod : Subsystem
  DesEquivRatio : Outport
  DFCOInfo : Outport  Port=2
  wires:
  EquivRatioInfo/1 -> Bus Selector/1
  Bus Selector/2 -> Bus Creator/2  "<WarmUpRatio>"
  Bus Selector/3 -> Bus Creator/3  "<WarmUptimeRatio>"
  Bus Creator/1 -> DesEquivRatio/1
  Sensors/1 -> DesEquivRatioMod/2(Sensors)
  DesEquivRatioMod/2(DFCOInfo) -> DFCOInfo/1
  Bus Selector/1 -> DesEquivRatioMod/1(DesEquivRatio_In)  "<DesEquivRatio>"
  DesEquivRatioMod/1(DesEquivRatio) -> Bus Creator/1  "DesEquivRatio"
  Bus Selector/4 -> Bus Creator/4  "<IATEnrichment>"
  Bus Selector/5 -> Bus Creator/5  "<CATEnrichment>"
